simulink model "q2"  (R2018b)
settings: Solver=VariableStepAuto  StartTime=0.0  StopTime=10.0  RelTol=1e-3
libraries: simulink x4
settings Model: Creator=Kasia  LastModifiedBy=Kasia

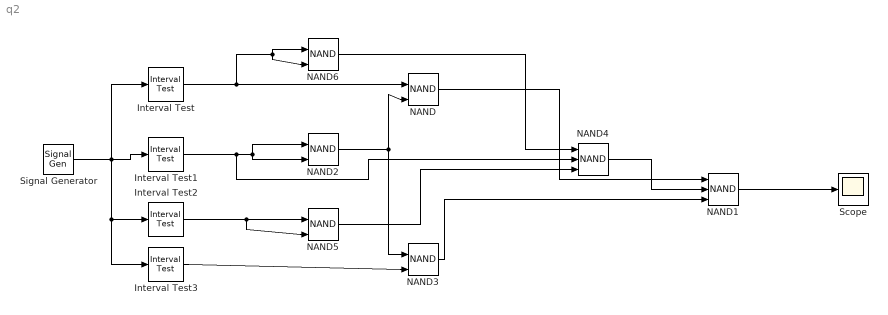
== system q2 ==
  Interval Test{,1..3} (4 alike) : simulink/Logic and Bit Operations/Interval Test  IntervalClosedRight=on  uplimit=0.5  IntervalClosedLeft=on  lowlimit=-0.5  OutDataTypeStr=boolean
  NAND{,2..3,5..6} (5 alike) : Logic  Operator=NAND  IconShape=distinctive  AllPortsSameDT=off  OutDataTypeStr=boolean
  NAND1 : Logic  Operator=NAND  Inputs=3  IconShape=distinctive  AllPortsSameDT=off  OutDataTypeStr=boolean
  NAND4 : Logic  Operator=NAND  Inputs=3  IconShape=distinctive  AllPortsSameDT=off  OutDataTypeStr=boolean
  Scope : Scope
  Signal Generator : SignalGenerator  Units=rad/sec
  wires:
  NAND/1 -> NAND1/1
  Interval Test1/1 -> NAND2/1, NAND2/2, NAND4/2
  NAND2/1 -> NAND3/1, NAND/2
  Interval Test3/1 -> NAND3/2
  NAND3/1 -> NAND1/3
  Signal Generator/1 -> Interval Test3/1, Interval Test2/1, Interval Test1/1, Interval Test/1
  NAND1/1 -> Scope/1
  Interval Test2/1 -> NAND5/2, NAND5/1
  NAND5/1 -> NAND4/3
  Interval Test/1 -> NAND/1, NAND6/1, NAND6/2
  NAND6/1 -> NAND4/1
  NAND4/1 -> NAND1/2
